simulink model "Three_Phase_VSG_Double_Loop_Control"  (R2024b)
settings: Solver=ode45  StartTime=0.0  StopTime=1.5  FixedStep=1e-4  RelTol=1e-3  EnableMultiTasking=on
libraries: powerlib_extras x11, spsGroundLib x3, spsThreePhaseSeriesRLCBranchLib x2, spsThreePhaseParallelRLCBranchLib x2, spsThreePhaseVIMeasurementLib x2, spsThreePhaseBreakerLib x2, spsDCVoltageSourceLib x1, spsPWMGenerator2LevelLib x1, spsUniversalBridgeLib x1, sps_lib x1
settings Model: SimulationMode=rapid-accelerator  Creator=hp  LastModifiedBy=27443
settings SolverCC: AlgebraicLoopSolver=TrustRegion
settings DataIOCC: LimitDataPoints=on  SaveFormat=Array  ReturnWorkspaceOutputs=off
settings OptimizationCC: LifeSpan=inf
settings DebuggingCC: SolverPrmCheckMsg=warning  UnconnectedInputMsg=warning  UnconnectedOutputMsg=warning  UnconnectedLineMsg=warning  SFUnexpectedBacktrackingDiag=warning  SFNoUnconditionalDefaultTransitionDiag=warning  SFExecutionAtInitializationDiag=none  ArithmeticOperatorsInVariantConditions=warning
settings HardwareCC: ProdBitPerPointer=32  ProdBitPerSizeT=32  ProdBitPerPtrDiffT=32  ProdLargestAtomicFloat=None  ProdIntDivRoundTo=Undefined  ProdEndianess=Unspecified  ProdWordSize=32  ProdHWDeviceType=32-bit Generic
settings ModelReferenceCC: EnableRefExpFcnMdlSchedulingChecks=on  PropagateSignalLabelsOutOfModel=off
settings SFSimCC: SimUseLocalCustomCode=off  CustomCodeUndefinedFunction=UseInterfaceOnly
settings RTWCC: RTWUseLocalCustomCode=off  GPUComputeCapability=3.5
settings CodeAppCC: StateflowObjectComments=on
settings GRTTargetCC: TargetLangStandard=C89/C90 (ANSI)
settings ConfigComp: CovMetricSettings=dw  CovSaveCumulativeToWorkspaceVar=on  CovSaveSingleToWorkspaceVar=on  CovExternalEMLEnable=off  CovSFcnEnable=off
settings SimscapeCC: SimscapeNormalizeSystem=off

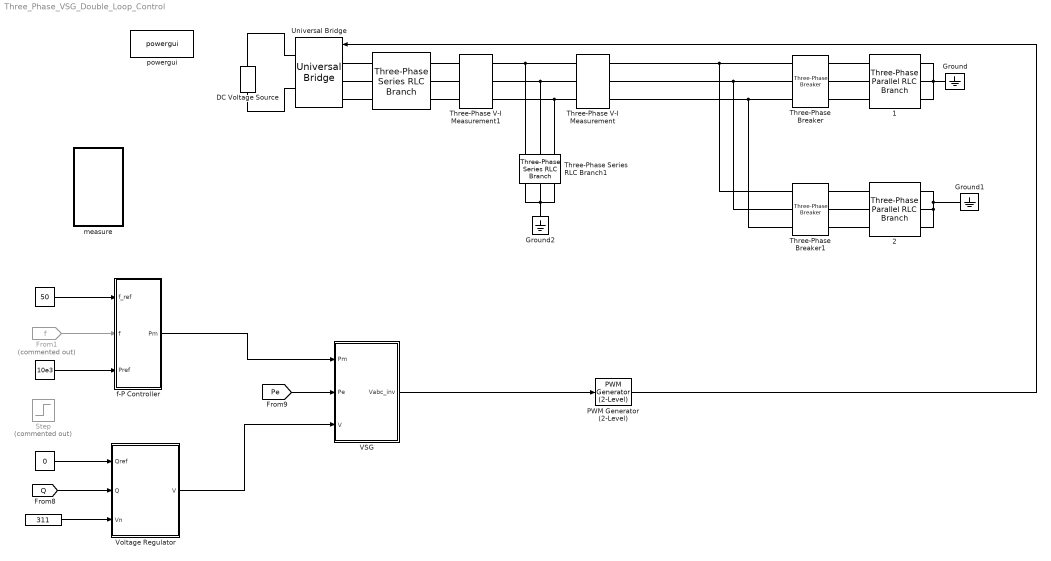
== system Three_Phase_VSG_Double_Loop_Control ==
  "         " : Constant  Value=50
  "           " : Constant  Value=10e3
  "             " : Constant  Value=0
  "               " : Constant  Value=311
  "                              " : spsThreePhaseSeriesRLCBranchLib/Three-Phase Series RLC Branch  LConnTagsString=A|B|C  RConnTagsString=A|B|C  BranchType=L  Resistance=0.01  Inductance=0.0184  Capacitance=1e-6  Measurements=None
  1 : spsThreePhaseParallelRLCBranchLib/Three-Phase Parallel RLC Branch  LConnTagsString=A|B|C  RConnTagsString=A|B|C  BranchType=R  Resistance=380^2/9844  Inductance=1e-3  Capacitance=1e-6  Measurements=None
  2 : spsThreePhaseParallelRLCBranchLib/Three-Phase Parallel RLC Branch  LConnTagsString=A|B|C  RConnTagsString=A|B|C  BranchType=R  Resistance=380^2/4e3  Inductance=1e-3  Capacitance=1e-6  Measurements=None
  DC Voltage Source : spsDCVoltageSourceLib/DC Voltage Source  Amplitude=800  Measurements=None
  From1 : From  Commented=on  GotoTag=f  TagVisibility=global
      settings: CloseFcn=tagdialog Close
  Ground : spsGroundLib/Ground  LConnTagsString=a
  Ground1 : spsGroundLib/Ground  LConnTagsString=a
  Ground2 : spsGroundLib/Ground  LConnTagsString=a
  PWM Generator (2-Level) : spsPWMGenerator2LevelLib/PWM Generator (2-Level)  ModulatorType=Three-phase bridge (6 pulses)  ModulatorMode=Unsynchronized  Fc=10000  Pc=90  nF=27  MinMax="[ -1  1 ]"  SamplingTechnique=Natural  ModulatingSignals=off  m=0.8  Freq=60  Phase=0  Ts=1e-6  ShowCarrierOutport=off
  Step : Step  Commented=on  Before=10000  After=12000  SampleTime=0
  Three-Phase Series RLC Branch1 : spsThreePhaseSeriesRLCBranchLib/Three-Phase Series RLC Branch  LConnTagsString=A|B|C  RConnTagsString=A|B|C  BranchType=C  Resistance=380^2 /10e3  Inductance=1e-3  Capacitance=10e-6  Measurements=None
  Three-Phase V-I Measurement : spsThreePhaseVIMeasurementLib/Three-Phase V-I Measurement  VoltageMeasurement=phase-to-ground  SetLabelV=on  LabelV=Vabc  Vpu=off  VpuLL=off  CurrentMeasurement=yes  SetLabelI=on  LabelI=Iabc  Ipu=off  Pbase=100e6  Vbase=380  OutputType=Complex  PhasorSimulation=off  PSBequivalent=0
  Three-Phase V-I Measurement1 : spsThreePhaseVIMeasurementLib/Three-Phase V-I Measurement  VoltageMeasurement=no  SetLabelV=off  LabelV=Vabc  Vpu=off  VpuLL=off  CurrentMeasurement=yes  SetLabelI=on  LabelI=Is_abc  Ipu=off  Pbase=100e6  Vbase=380  OutputType=Complex  PhasorSimulation=off  PSBequivalent=0
  Three-Phase Breaker : spsThreePhaseBreakerLib/Three-Phase Breaker  InitialState=closed  SwitchA=on  SwitchB=on  SwitchC=on  SwitchTimes="[4/60  10/60]+100"  External=off  BreakerResistance=0.001  SnubberResistance=1e6  SnubberCapacitance=inf  Measurements=None
  Three-Phase Breaker1 : spsThreePhaseBreakerLib/Three-Phase Breaker  InitialState=open  SwitchA=on  SwitchB=on  SwitchC=on  SwitchTimes="[0.4  0.8]"  External=off  BreakerResistance=0.001  SnubberResistance=1e6  SnubberCapacitance=inf  Measurements=None
  Universal Bridge : spsUniversalBridgeLib/Universal Bridge  Arms=3  SnubberResistance=1e5  SnubberCapacitance=inf  Device=IGBT / Diodes  Ron=1e-3  Lon=0  ForwardVoltages="[  0  0  ]"  ForwardVoltage=0  GTOparameters=[ 10e-6 , 20e-6 ]  IGBTparameters=[ 1e-6 , 2e-6 ]  Measurements=None  Measurements_2=None  converterType=Rectifier
  VSG : Subsystem
  Voltage Regulator : Subsystem
  f-P Controller : Subsystem
  measure : Subsystem
  powergui : sps_lib/powergui  SimulationMode=Discrete  SampleTime=1e-6  frequency=60  Iterations=50  frequencyindice=0  Pbase=100e6  ErrMax=1e-4  UnitsV=kV  UnitsW=MW  buscounter=0  FunctionMessages=off  echomessages=off  EnableUseOfTLC=off  CurrentSourceSwitches=off  DisableSnubberDevices=off  DisableRonSwitches=off  DisableVfSwitches=off  DisplayEquations=off  AutomaticDiscreteSolvers=off  SolverType=Tustin  Interpol=off  ExternalGateDelay=off  methode=off  Ts=0  x0status=blocks  SPID=off  SwTol=0  HookPort=off  NonlinearTolerance=1e-4  nMaxIteration=100  ContinueOnMaxIteration=off  RestoreLinks=warning  ResistiveCurrentMeasurement=off  Frange=[0:2:500]  Ylog=off  Xlog=on  ShowGrid=off  save=off  variable=ZData  structure=ScopeData6  ZoomFFT=on  StartTime=2.0  cycles=5  DisplayStyle=2  fundamental=50  FreqAxis=on  MaxFrequency=500  frequencyindicesteady=1  RmsSteady=1  display=off
  wires:
  "         "/1 -> f-P Controller/1(f_ref)
  "               "/1 -> Voltage Regulator/3(Vn)
  From1/1 -> f-P Controller/2(f)
  "             "/1 -> Voltage Regulator/1(Qref)
  [Q] -> Voltage Regulator/2(Q)
  [Pe] -> VSG/2(Pe)
  Voltage Regulator/1(V) -> VSG/3(V)
  f-P Controller/1(Pm) -> VSG/1(Pm)
  PWM Generator (2-Level)/1 -> Universal Bridge/1
  VSG/1(Vabc_inv) -> PWM Generator (2-Level)/1
  "           "/1 -> f-P Controller/3(Pref)
  connections:
  Three-Phase V-I Measurement/LConn3 -- Three-Phase V-I Measurement1/RConn3 -- Three-Phase Series RLC Branch1/LConn3
  Three-Phase V-I Measurement/LConn2 -- Three-Phase V-I Measurement1/RConn2 -- Three-Phase Series RLC Branch1/LConn2
  Three-Phase V-I Measurement/LConn1 -- Three-Phase V-I Measurement1/RConn1 -- Three-Phase Series RLC Branch1/LConn1
  Three-Phase Series RLC Branch1/RConn2 -- Ground2/LConn1 -- Three-Phase Series RLC Branch1/RConn1 -- Three-Phase Series RLC Branch1/RConn3
  Three-Phase Breaker1/LConn1 -- Three-Phase Breaker/LConn1 -- Three-Phase V-I Measurement/RConn1
  Three-Phase Breaker1/LConn2 -- Three-Phase Breaker/LConn2 -- Three-Phase V-I Measurement/RConn2
  Three-Phase Breaker/LConn3 -- Three-Phase Breaker1/LConn3 -- Three-Phase V-I Measurement/RConn3
  Ground/LConn1 -- 1/RConn1 -- 1/RConn3 -- 1/RConn2
  Ground1/LConn1 -- 2/RConn1 -- 2/RConn3 -- 2/RConn2
  DC Voltage Source/RConn1 -- Universal Bridge/RConn1
  Universal Bridge/LConn1 -- "                              "/LConn1
  Three-Phase Breaker/RConn1 -- 1/LConn1
  Universal Bridge/RConn2 -- DC Voltage Source/LConn1
  Universal Bridge/LConn2 -- "                              "/LConn2
  Universal Bridge/LConn3 -- "                              "/LConn3
  Three-Phase Breaker/RConn3 -- 1/LConn3
  Three-Phase Breaker1/RConn3 -- 2/LConn3
  Three-Phase Breaker1/RConn1 -- 2/LConn1
  Three-Phase Breaker1/RConn2 -- 2/LConn2
  Three-Phase Breaker/RConn2 -- 1/LConn2
  Three-Phase V-I Measurement1/LConn1 -- "                              "/RConn1
  Three-Phase V-I Measurement1/LConn2 -- "                              "/RConn2
  Three-Phase V-I Measurement1/LConn3 -- "                              "/RConn3

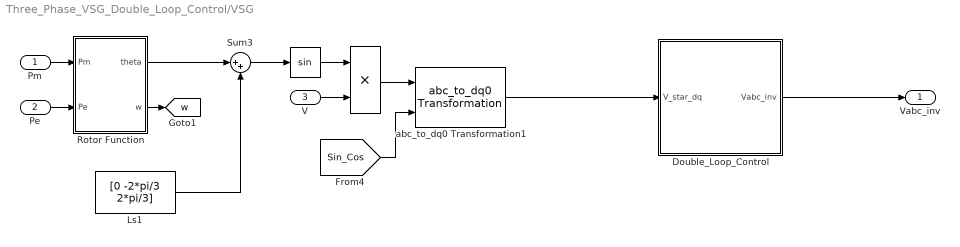
== system Three_Phase_VSG_Double_Loop_Control/VSG ==
  Pm : Inport
  Pe : Inport  Port=2
  V : Inport  Port=3
  " " : Trigonometry
  "  " : Product
  Double_Loop_Control : Subsystem
  Ls1 : Constant  Value=[0 -2*pi/3 2*pi/3]
  Rotor Function : Subsystem
  Sum3 : Sum  Inputs=|++
  abc_to_dq0 Transformation1 : powerlib_extras/Measurements/abc_to_dq0 Transformation
  Vabc_inv : Outport  VectorParamsAs1DForOutWhenUnconnected=off
  tag scope: w=global
  wires:
  " "/1 -> "  "/1
  Pe/1 -> Rotor Function/2(Pe)
  Pm/1 -> Rotor Function/1(Pm)
  V/1 -> "  "/2
  Ls1/1 -> Sum3/2
  Sum3/1 -> " "/1
  Rotor Function/1(theta) -> Sum3/1
  [Sin_Cos] -> abc_to_dq0 Transformation1/2
  "  "/1 -> abc_to_dq0 Transformation1/1
  Rotor Function/2(w) -> [w]
  abc_to_dq0 Transformation1/1 -> Double_Loop_Control/1(V_star_dq)
  Double_Loop_Control/1(Vabc_inv) -> Vabc_inv/1

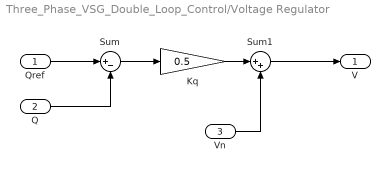
== system Three_Phase_VSG_Double_Loop_Control/Voltage Regulator ==
  Qref : Inport
  Q : Inport  Port=2
  Vn : Inport  Port=3
  Kq : Gain  Gain=0.5
  Sum : Sum  Inputs=|+-
  Sum1 : Sum  Inputs=|++
  V : Outport  VectorParamsAs1DForOutWhenUnconnected=off
  wires:
  Sum1/1 -> V/1
  Kq/1 -> Sum1/1
  Qref/1 -> Sum/1
  Q/1 -> Sum/2
  Vn/1 -> Sum1/2
  Sum/1 -> Kq/1

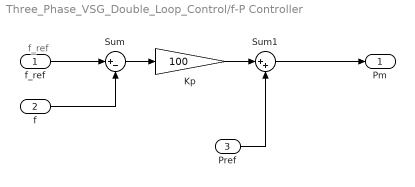
== system Three_Phase_VSG_Double_Loop_Control/f-P Controller ==
  note: f_ref
  f_ref : Inport
  f : Inport  Port=2
  Pref : Inport  Port=3
  Kp : Gain  Gain=100
  Sum : Sum  Inputs=|+-
  Sum1 : Sum  Inputs=|++
  Pm : Outport  VectorParamsAs1DForOutWhenUnconnected=off
  wires:
  Sum1/1 -> Pm/1
  Sum/1 -> Kp/1
  Pref/1 -> Sum1/2
  f/1 -> Sum/2
  f_ref/1 -> Sum/1
  Kp/1 -> Sum1/1

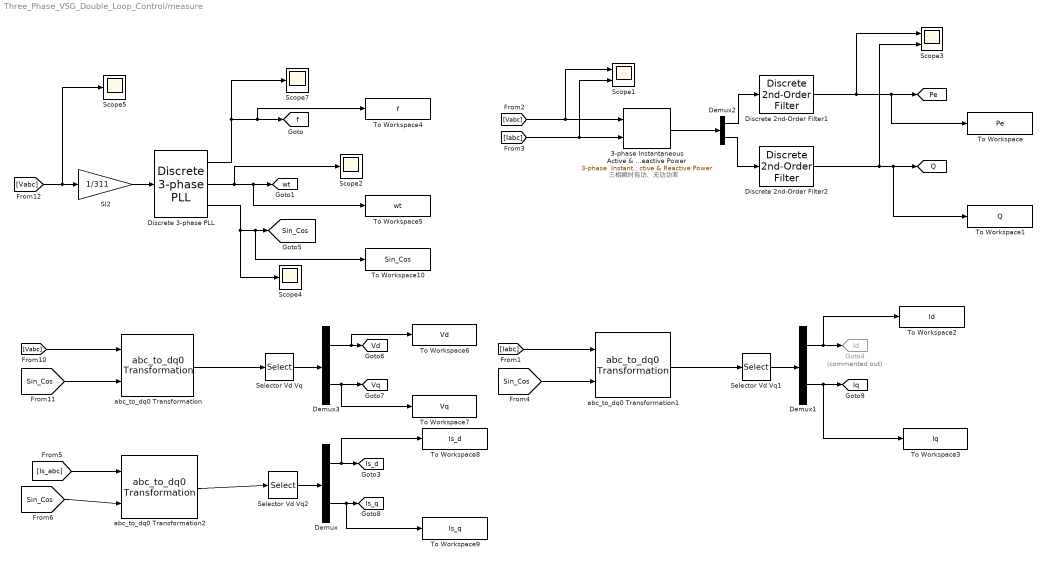
== system Three_Phase_VSG_Double_Loop_Control/measure ==
  note: 三相瞬时有功、无功功率
  3-phase Instantaneous Active & Reactive Power : powerlib_extras/Measurements/3-phase  Instantaneous  Active & Reactive Power
  Demux{,1..3} (4 alike) : Demux  Outputs=2
  Discrete 2nd-Order Filter1 : powerlib_extras/Discrete  Control Blocks/Discrete  2nd-Order Filter  FilterType=Lowpass  Fo=1000  Zeta=0.707  Ts=5e-6  Initialize=off  Vac_Init=[0.8 -25 60]  Vdc_Init=-0.4  PlotResponse=off  param1=[1 500 1]
  Discrete 2nd-Order Filter2 : powerlib_extras/Discrete  Control Blocks/Discrete  2nd-Order Filter  FilterType=Lowpass  Fo=1000  Zeta=0.707  Ts=5e-6  Initialize=off  Vac_Init=[0.8 -25 60]  Vdc_Init=-0.4  PlotResponse=off  param1=[1 500 1]
  Discrete 3-phase PLL : powerlib_extras/Discrete  Control Blocks/Discrete 3-phase PLL  Fmin=45  Par_Init=[0 50]  ParK=[0.001 0.005 0]  Ts=1e-6  AGC=off
  Goto4 : Goto  Commented=on  GotoTag=Id  TagVisibility=global
  SI2 : Gain  Gain=1/311
  Scope1 : Scope  NumInputPorts=2
  Scope{2,4..5,7} (4 alike) : Scope
  Scope3 : Scope  NumInputPorts=2
  Selector Vd Vq : Selector  InputPortWidth=3  IndexOptions=Index vector (dialog)  Indices=[1 2]  OutputSizes=1
  Selector Vd Vq1 : Selector  InputPortWidth=3  IndexOptions=Index vector (dialog)  Indices=[1 2]  OutputSizes=1
  Selector Vd Vq2 : Selector  InputPortWidth=3  IndexOptions=Index vector (dialog)  Indices=[1 2]  OutputSizes=1
  To Workspace : ToWorkspace  VariableName=Pe  SaveFormat=Timeseries  SampleTime=-1
  To Workspace1 : ToWorkspace  VariableName=Q  SaveFormat=Timeseries  SampleTime=-1
  To Workspace10 : ToWorkspace  VariableName=Sin_Cos  SaveFormat=Timeseries  SampleTime=-1
  To Workspace2 : ToWorkspace  VariableName=Id  SaveFormat=Timeseries  SampleTime=-1
  To Workspace3 : ToWorkspace  VariableName=Iq  SaveFormat=Timeseries  SampleTime=-1
  To Workspace4 : ToWorkspace  VariableName=f  SaveFormat=Timeseries  SampleTime=-1
  To Workspace5 : ToWorkspace  VariableName=wt  SaveFormat=Timeseries  SampleTime=-1
  To Workspace6 : ToWorkspace  VariableName=Vd  SaveFormat=Timeseries  SampleTime=-1
  To Workspace7 : ToWorkspace  VariableName=Vq  SaveFormat=Timeseries  SampleTime=-1
  To Workspace8 : ToWorkspace  VariableName=Is_d  SaveFormat=Timeseries  SampleTime=-1
  To Workspace9 : ToWorkspace  VariableName=Is_q  SaveFormat=Timeseries  SampleTime=-1
  abc_to_dq0 Transformation : powerlib_extras/Measurements/abc_to_dq0 Transformation
  abc_to_dq0 Transformation1 : powerlib_extras/Measurements/abc_to_dq0 Transformation
  abc_to_dq0 Transformation2 : powerlib_extras/Measurements/abc_to_dq0 Transformation
  tag scope: Iq=global, Is_d=global, Is_q=global, Pe=global, Q=global, Sin_Cos=global, Vd=global, Vq=global, f=global, wt=global
  wires:
  [Vabc] -> Scope5/1, SI2/1
  Discrete 3-phase PLL/1 -> Scope7/1, To Workspace4/1, [f]
  [Iabc] -> 3-phase Instantaneous Active & Reactive Power/2, Scope1/2
  [Vabc] -> abc_to_dq0 Transformation/1
  Discrete 3-phase PLL/3 -> Scope4/1, To Workspace10/1, [Sin_Cos]
  Discrete 3-phase PLL/2 -> Scope2/1, To Workspace5/1, [wt]
  Demux2/1 -> Discrete 2nd-Order Filter1/1
  [Sin_Cos] -> abc_to_dq0 Transformation/2
  abc_to_dq0 Transformation/1 -> Selector Vd Vq/1
  SI2/1 -> Discrete 3-phase PLL/1
  Demux2/2 -> Discrete 2nd-Order Filter2/1
  [Vabc] -> 3-phase Instantaneous Active & Reactive Power/1, Scope1/1
  3-phase Instantaneous Active & Reactive Power/1 -> Demux2/1
  Discrete 2nd-Order Filter1/1 -> Scope3/1, To Workspace/1, [Pe]
  Discrete 2nd-Order Filter2/1 -> To Workspace1/1, [Q], Scope3/2
  [Sin_Cos] -> abc_to_dq0 Transformation1/2
  [Iabc] -> abc_to_dq0 Transformation1/1
  abc_to_dq0 Transformation1/1 -> Selector Vd Vq1/1
  [Sin_Cos] -> abc_to_dq0 Transformation2/2
  abc_to_dq0 Transformation2/1 -> Selector Vd Vq2/1
  [Is_abc] -> abc_to_dq0 Transformation2/1
  Selector Vd Vq/1 -> Demux3/1
  Demux3/1 -> To Workspace6/1, [Vd]
  Demux3/2 -> To Workspace7/1, [Vq]
  Selector Vd Vq2/1 -> Demux/1
  Demux/1 -> To Workspace8/1, [Is_d]
  Demux/2 -> To Workspace9/1, [Is_q]
  Selector Vd Vq1/1 -> Demux1/1
  Demux1/1 -> To Workspace2/1, Goto4/1
  Demux1/2 -> To Workspace3/1, [Iq]

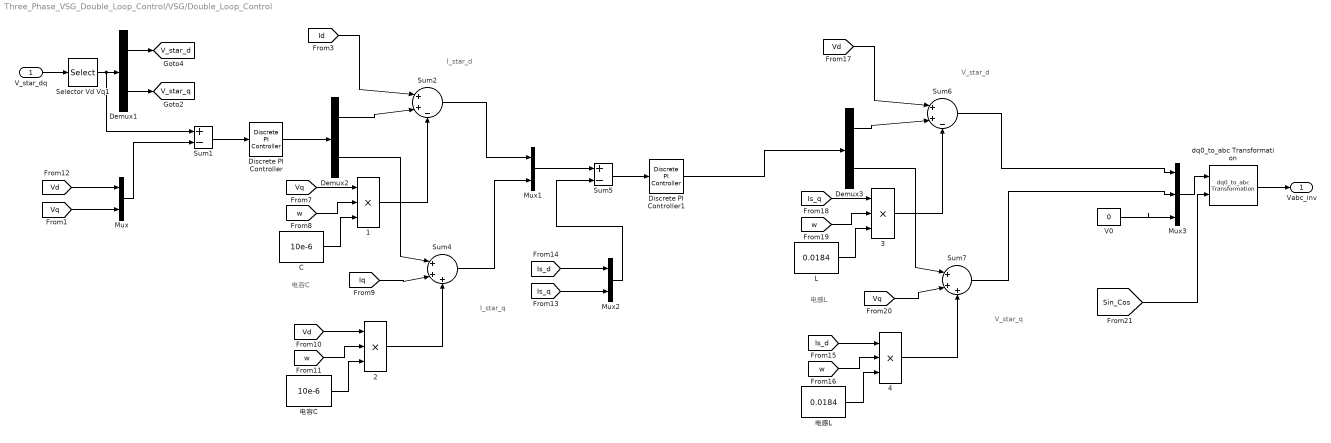
== system Three_Phase_VSG_Double_Loop_Control/VSG/Double_Loop_Control ==
  note: 电感L
  note: 电容C
  note: I_star_q
  note: I_star_d
  note: V_star_q
  note: V_star_d
  V_star_dq : Inport
    {1..4} (4 alike) : Product  Inputs=3
  C : Constant  Value=10e-6
  Demux1 : Demux  Outputs=2
  Demux2 : Demux  Outputs=2
  Demux3 : Demux  Outputs=2
  Discrete PI Controller : powerlib_extras/Discrete  Control Blocks/Discrete PI Controller  Kp=6  Ki=1  Par_Limits=[1000 -1000]  Init=0  Ts=1e-6
  Discrete PI Controller1 : powerlib_extras/Discrete  Control Blocks/Discrete PI Controller  Kp=5  Ki=1  Par_Limits=[1000 -1000]  Init=0  Ts=1e-6
  L : Constant  Value=0.0184
  Mux : Mux  Inputs=2
  Mux1 : Mux  Inputs=2
  Mux2 : Mux  Inputs=2
  Mux3 : Mux  Inputs=3
  Selector Vd Vq1 : Selector  InputPortWidth=3  IndexOptions=Index vector (dialog)  Indices=[1 2]  OutputSizes=1
  Sum1 : Sum  Inputs=+-  InputSameDT=on  SaturateOnIntegerOverflow=on  OutDataTypeStr=Inherit: Same as first input
  Sum2 : Sum  Inputs=|++-
  Sum4 : Sum  Inputs=|+++
  Sum5 : Sum  Inputs=+-  InputSameDT=on  SaturateOnIntegerOverflow=on  OutDataTypeStr=Inherit: Same as first input
  Sum6 : Sum  Inputs=|++-
  Sum7 : Sum  Inputs=|+++
  V0 : Constant  Value=0
  dq0_to_abc Transformation : powerlib_extras/Measurements/dq0_to_abc Transformation
  电容C : Constant  Value=10e-6
  电感L : Constant  Value=0.0184
  Vabc_inv : Outport  VectorParamsAs1DForOutWhenUnconnected=off
  tag scope: V_star_d=global, V_star_q=global
  wires:
  [Is_q] -> Mux2/2
  [Vq] -> "  1"/1
  V0/1 -> Mux3/3
  Mux3/1 -> dq0_to_abc Transformation/1
  Demux1/1 -> [V_star_d]
  Sum6/1 -> Mux3/1
  dq0_to_abc Transformation/1 -> Vabc_inv/1
  "  1"/1 -> Sum2/3
  Demux1/2 -> [V_star_q]
  Sum2/1 -> Mux1/1
  [Id] -> Sum2/1
  Sum7/1 -> Mux3/2
  Mux2/1 -> Sum5/2
  [Is_d] -> Mux2/1
  电感L/1 -> "  4"/3
  Demux2/2 -> Sum4/1
  Mux1/1 -> Sum5/1
  [Sin_Cos] -> dq0_to_abc Transformation/2
  Mux/1 -> Sum1/2
  [w] -> "  4"/2
  [Is_d] -> "  4"/1
  Sum4/1 -> Mux1/2
  Discrete PI Controller/1 -> Demux2/1
  [Iq] -> Sum4/2
  [w] -> "  1"/2
  Demux2/1 -> Sum2/2
  [w] -> "  2"/2
  Sum5/1 -> Discrete PI Controller1/1
  [Vq] -> Mux/2
  Discrete PI Controller1/1 -> Demux3/1
  "  2"/1 -> Sum4/3
  [Vd] -> "  2"/1
  [Is_q] -> "  3"/1
  L/1 -> "  3"/3
  Demux3/1 -> Sum6/2
  Demux3/2 -> Sum7/1
  C/1 -> "  1"/3
  [Vd] -> Sum6/1
  [Vq] -> Sum7/2
  Selector Vd Vq1/1 -> Sum1/1, Demux1/1
  [w] -> "  3"/2
  "  4"/1 -> Sum7/3
  "  3"/1 -> Sum6/3
  [Vd] -> Mux/1
  电容C/1 -> "  2"/3
  Sum1/1 -> Discrete PI Controller/1
  V_star_dq/1 -> Selector Vd Vq1/1

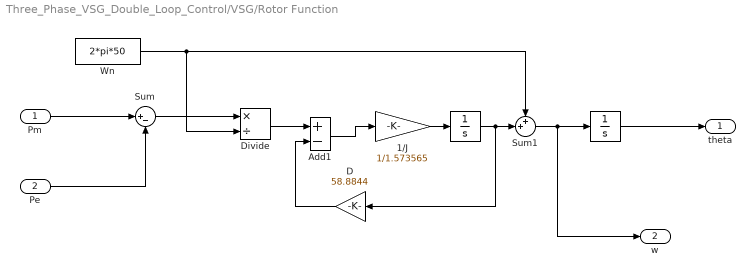
== system Three_Phase_VSG_Double_Loop_Control/VSG/Rotor Function ==
  Pm : Inport
  Pe : Inport  Port=2
  " " : Integrator  LimitOutput=on  UpperSaturationLimit=2*pi*0.5  LowerSaturationLimit=-2*pi*0.5
  "    " : Integrator
  1/J : Gain  Gain=1/1.573565
  Add1 : Sum  Inputs=+-
  D : Gain  Gain=58.8844
  Divide : Product  Inputs=*/
  Sum : Sum  Inputs=|+-
  Sum1 : Sum  Inputs=++|
  Wn : Constant  Value=2*pi*50
  theta : Outport  VectorParamsAs1DForOutWhenUnconnected=off
  w : Outport  Port=2  VectorParamsAs1DForOutWhenUnconnected=off
  wires:
  Sum1/1 -> w/1, "    "/1
  Wn/1 -> Sum1/1, Divide/2
  1/J/1 -> " "/1
  Pm/1 -> Sum/1
  "    "/1 -> theta/1
  Pe/1 -> Sum/2
  Sum/1 -> Divide/1
  D/1 -> Add1/2
  " "/1 -> D/1, Sum1/2
  Divide/1 -> Add1/1
  Add1/1 -> 1/J/1
